simulink model "THREE_PID"  (R2019b)
settings: Solver=ode45  StartTime=0.0  StopTime=5  MaxStep=0.5  MinStep=0.00001  RelTol=0.05
model workspace: external: MAT-File workspace.mat (data not in the file)
values from neighbouring files (symbols this model uses):
  b = b+nb(i)    [genetic_pid.m]
  R = rand    [genetic_pid.m]
undefined symbols (not defined in the file or in its folder): B, F, g, GR, J1, J_rotor, k, km, kt, L, L1, L1C, M1
libraries: simulink x3, simulink_extras x3
settings Model: Creator=Kartik  LastModifiedBy=Kartik
settings SolverCC: MaxConsecutiveMinStep=20  ZeroCrossAlgorithm=Adaptive
settings DataIOCC: Refine=2
settings DebuggingCC: MaskedZcDiagnostic=none  IgnoredZcDiagnostic=none

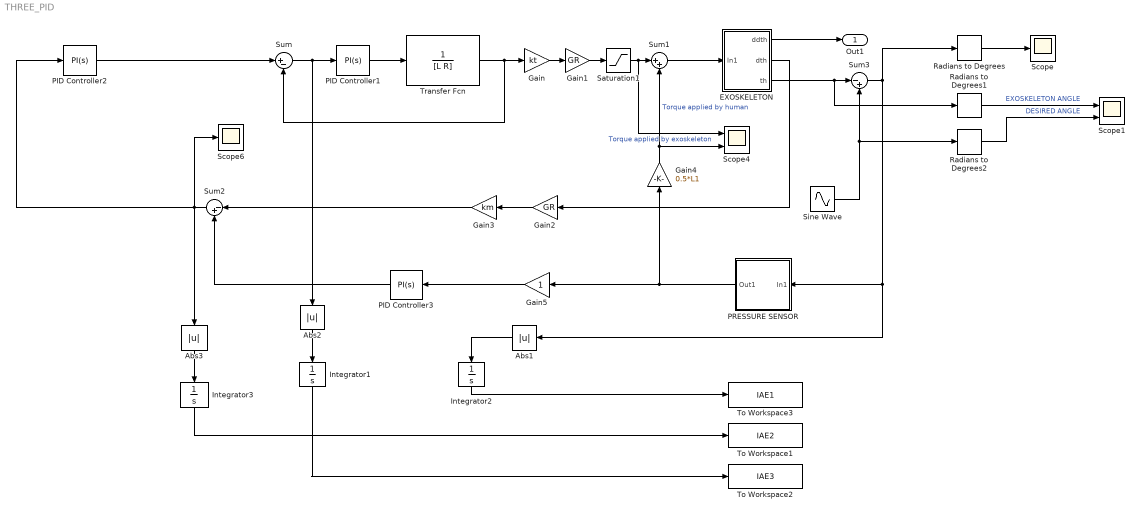
== system THREE_PID ==
  Abs1 : Abs
  Abs2 : Abs
  Abs3 : Abs
  "EXOSKELETON " : Subsystem
  Gain : Gain  Gain=kt
  Gain1 : Gain  Gain=GR
  Gain2 : Gain  Gain=GR
  Gain3 : Gain  Gain=km
  Gain4 : Gain  Gain=0.5*L1
  Gain5 : Gain
  Integrator1 : Integrator
  Integrator2 : Integrator
  Integrator3 : Integrator
  PID Controller1 : simulink/Continuous/PID Controller  Controller=PI  Form=Parallel  TimeDomain=Continuous-time  SampleTime=-1  IntegratorMethod=Forward Euler  FilterMethod=Forward Euler  ControllerParametersSource=internal  P=13.44220  I=9.960331  D=0  UseFilter=on  N=100  TunerSelectOption=Transfer Function Based (PID Tuner App)  InitialConditionSource=internal  InitialConditionForIntegrator=0  InitialConditionForFilter=0  DifferentiatorICPrevScaledInput=0  ExternalReset=none  TrackingMode=off  Kt=1  LimitOutput=off  UpperSaturationLimit=inf  LowerSaturationLimit=-inf  LinearizeAsGain=on  AntiWindupMode=none  Kb=1  POutMin=[]  POutMax=[]  IOutMin=[]  IOutMax=[]  DOutMin=[]  DOutMax=[]  NOutMin=[]  NOutMax=[]  SumOutMin=[]  SumOutMax=[]  SaturationOutMin=[]  SaturationOutMax=[]  PParamMin=[]  PParamMax=[]  IParamMin=[]  IParamMax=[]  DParamMin=[]  DParamMax=[]  NParamMin=[]  NParamMax=[]  KbParamMin=[]  KbParamMax=[]  KtParamMin=[]  KtParamMax=[]  KbOutMin=[]  KbOutMax=[]  KtOutMin=[]  KtOutMax=[]  IntegratorOutMin=[]  IntegratorOutMax=[]  FilterOutMin=[]  FilterOutMax=[]  SumI1OutMin=[]  SumI1OutMax=[]  SumI2OutMin=[]  SumI2OutMax=[]  SumI3OutMin=[]  SumI3OutMax=[]  SumI4OutMin=[]  SumI4OutMax=[]  SumDOutMin=[]  SumDOutMax=[]  DifferentiatorOutMin=[]  DifferentiatorOutMax=[]  FilterDiffOutCoefMin=[]  FilterDiffOutCoefMax=[]  ReciprocalOutMin=[]  ReciprocalOutMax=[]  SumDenOutMin=[]  SumDenOutMax=[]  SumNumOutMin=[]  SumNumOutMax=[]  DivideOutMin=[]  DivideOutMax=[]  IntegratorContinuousStateAttributes=''  IntegratorStateMustResolveToSignalObject=off  IntegratorRTWStateStorageClass=Auto  FilterContinuousStateAttributes=''  FilterStateMustResolveToSignalObject=off  FilterRTWStateStorageClass=Auto  ParallelPVariant=InternalParameters  IdealPVariant=Disabled  IVariant=InternalParameters  DVariant=Disabled  IntegratorVariant=Continuous  SatVariant=Disabled  AWVariant=Passthrough  PCopyVariant=Disabled  TRVariant=Disabled  FdbkBlocksVariant=Forward  IdealPFdbkVariant=Disabled  SatFdbkVariant=Disabled  DerivativeFilterVariant=Disabled  NVariant=Disabled  NCopyVariant=Disabled_SignalSpec  FilterICVariant=Disabled  IntegratorICVariant=InternalICs  ExternalResetVariant=Disabled  TRSumVariant=Passthrough  SumFdbkVariant=Disabled  SumVariant=Sum_PI
  PID Controller2 : simulink/Continuous/PID Controller  Controller=PI  Form=Parallel  TimeDomain=Continuous-time  SampleTime=-1  IntegratorMethod=Forward Euler  FilterMethod=Forward Euler  ControllerParametersSource=internal  P=1.611515  I=1.022319  D=0  UseFilter=on  N=100  TunerSelectOption=Transfer Function Based (PID Tuner App)  InitialConditionSource=internal  InitialConditionForIntegrator=0  InitialConditionForFilter=0  DifferentiatorICPrevScaledInput=0  ExternalReset=none  TrackingMode=off  Kt=1  LimitOutput=off  UpperSaturationLimit=inf  LowerSaturationLimit=-inf  LinearizeAsGain=on  AntiWindupMode=none  Kb=1  POutMin=[]  POutMax=[]  IOutMin=[]  IOutMax=[]  DOutMin=[]  DOutMax=[]  NOutMin=[]  NOutMax=[]  SumOutMin=[]  SumOutMax=[]  SaturationOutMin=[]  SaturationOutMax=[]  PParamMin=[]  PParamMax=[]  IParamMin=[]  IParamMax=[]  DParamMin=[]  DParamMax=[]  NParamMin=[]  NParamMax=[]  KbParamMin=[]  KbParamMax=[]  KtParamMin=[]  KtParamMax=[]  KbOutMin=[]  KbOutMax=[]  KtOutMin=[]  KtOutMax=[]  IntegratorOutMin=[]  IntegratorOutMax=[]  FilterOutMin=[]  FilterOutMax=[]  SumI1OutMin=[]  SumI1OutMax=[]  SumI2OutMin=[]  SumI2OutMax=[]  SumI3OutMin=[]  SumI3OutMax=[]  SumI4OutMin=[]  SumI4OutMax=[]  SumDOutMin=[]  SumDOutMax=[]  DifferentiatorOutMin=[]  DifferentiatorOutMax=[]  FilterDiffOutCoefMin=[]  FilterDiffOutCoefMax=[]  ReciprocalOutMin=[]  ReciprocalOutMax=[]  SumDenOutMin=[]  SumDenOutMax=[]  SumNumOutMin=[]  SumNumOutMax=[]  DivideOutMin=[]  DivideOutMax=[]  IntegratorContinuousStateAttributes=''  IntegratorStateMustResolveToSignalObject=off  IntegratorRTWStateStorageClass=Auto  FilterContinuousStateAttributes=''  FilterStateMustResolveToSignalObject=off  FilterRTWStateStorageClass=Auto  ParallelPVariant=InternalParameters  IdealPVariant=Disabled  IVariant=InternalParameters  DVariant=Disabled  IntegratorVariant=Continuous  SatVariant=Disabled  AWVariant=Passthrough  PCopyVariant=Disabled  TRVariant=Disabled  FdbkBlocksVariant=Forward  IdealPFdbkVariant=Disabled  SatFdbkVariant=Disabled  DerivativeFilterVariant=Disabled  NVariant=Disabled  NCopyVariant=Disabled_SignalSpec  FilterICVariant=Disabled  IntegratorICVariant=InternalICs  ExternalResetVariant=Disabled  TRSumVariant=Passthrough  SumFdbkVariant=Disabled  SumVariant=Sum_PI
  PID Controller3 : simulink/Continuous/PID Controller  Controller=PI  Form=Parallel  TimeDomain=Continuous-time  SampleTime=-1  IntegratorMethod=Forward Euler  FilterMethod=Forward Euler  ControllerParametersSource=internal  P=35.80372  I=4.633430  D=0  UseFilter=on  N=100  TunerSelectOption=Transfer Function Based (PID Tuner App)  InitialConditionSource=internal  InitialConditionForIntegrator=0  InitialConditionForFilter=0  DifferentiatorICPrevScaledInput=0  ExternalReset=none  TrackingMode=off  Kt=1  LimitOutput=off  UpperSaturationLimit=inf  LowerSaturationLimit=-inf  LinearizeAsGain=on  AntiWindupMode=none  Kb=1  POutMin=[]  POutMax=[]  IOutMin=[]  IOutMax=[]  DOutMin=[]  DOutMax=[]  NOutMin=[]  NOutMax=[]  SumOutMin=[]  SumOutMax=[]  SaturationOutMin=[]  SaturationOutMax=[]  PParamMin=[]  PParamMax=[]  IParamMin=[]  IParamMax=[]  DParamMin=[]  DParamMax=[]  NParamMin=[]  NParamMax=[]  KbParamMin=[]  KbParamMax=[]  KtParamMin=[]  KtParamMax=[]  KbOutMin=[]  KbOutMax=[]  KtOutMin=[]  KtOutMax=[]  IntegratorOutMin=[]  IntegratorOutMax=[]  FilterOutMin=[]  FilterOutMax=[]  SumI1OutMin=[]  SumI1OutMax=[]  SumI2OutMin=[]  SumI2OutMax=[]  SumI3OutMin=[]  SumI3OutMax=[]  SumI4OutMin=[]  SumI4OutMax=[]  SumDOutMin=[]  SumDOutMax=[]  DifferentiatorOutMin=[]  DifferentiatorOutMax=[]  FilterDiffOutCoefMin=[]  FilterDiffOutCoefMax=[]  ReciprocalOutMin=[]  ReciprocalOutMax=[]  SumDenOutMin=[]  SumDenOutMax=[]  SumNumOutMin=[]  SumNumOutMax=[]  DivideOutMin=[]  DivideOutMax=[]  IntegratorContinuousStateAttributes=''  IntegratorStateMustResolveToSignalObject=off  IntegratorRTWStateStorageClass=Auto  FilterContinuousStateAttributes=''  FilterStateMustResolveToSignalObject=off  FilterRTWStateStorageClass=Auto  ParallelPVariant=InternalParameters  IdealPVariant=Disabled  IVariant=InternalParameters  DVariant=Disabled  IntegratorVariant=Continuous  SatVariant=Disabled  AWVariant=Passthrough  PCopyVariant=Disabled  TRVariant=Disabled  FdbkBlocksVariant=Forward  IdealPFdbkVariant=Disabled  SatFdbkVariant=Disabled  DerivativeFilterVariant=Disabled  NVariant=Disabled  NCopyVariant=Disabled_SignalSpec  FilterICVariant=Disabled  IntegratorICVariant=InternalICs  ExternalResetVariant=Disabled  TRSumVariant=Passthrough  SumFdbkVariant=Disabled  SumVariant=Sum_PI
  PRESSURE SENSOR : Subsystem
  Radians to Degrees : simulink_extras/Transformations/Radians to Degrees
  Radians to Degrees1 : simulink_extras/Transformations/Radians to Degrees
  Radians to Degrees2 : simulink_extras/Transformations/Radians to Degrees
  Saturation1 : Saturate  UpperLimit=200  LowerLimit=-200
  Scope : Scope
  Scope1 : Scope  NumInputPorts=2
  Scope4 : Scope  NumInputPorts=2
  Scope6 : Scope
  Sine Wave : Sin  Amplitude=0.4  Frequency=2  SampleTime=0
  Sum : Sum  Inputs=|+-
  Sum1 : Sum  Inputs=|++
  Sum2 : Sum  Inputs=|-+
  Sum3 : Sum  Inputs=|-+
  To Workspace1 : ToWorkspace  VariableName=IAE2  SampleTime=-1
  To Workspace2 : ToWorkspace  VariableName=IAE3  SampleTime=-1
  To Workspace3 : ToWorkspace  VariableName=IAE1  SampleTime=-1
  Transfer Fcn : TransferFcn  Denominator=[L R]
  Out1 : Outport
  wires:
  PID Controller1/1 -> Transfer Fcn/1
  Sum/1 -> Abs2/1, PID Controller1/1
  PID Controller2/1 -> Sum/1
  Transfer Fcn/1 -> Gain/1, Sum/2
  Gain/1 -> Gain1/1
  "EXOSKELETON "/2(dth) -> Gain2/1
  Gain2/1 -> Gain3/1
  Gain3/1 -> Sum2/1
  "EXOSKELETON "/3(th) -> Radians to Degrees1/1, Sum3/1
  Sum3/1 -> Radians to Degrees/1, Abs1/1, PRESSURE SENSOR/1(In1)
  Gain4/1 -> Sum1/2, Scope4/2  "Torque applied by human"
  PID Controller3/1 -> Sum2/2
  "EXOSKELETON "/1(ddth) -> Out1/1
  Radians to Degrees/1 -> Scope/1
  Radians to Degrees1/1 -> Scope1/1  "EXOSKELETON ANGLE"
  Radians to Degrees2/1 -> Scope1/2  "DESIRED ANGLE"
  Abs1/1 -> Integrator2/1
  Integrator2/1 -> To Workspace3/1
  Gain5/1 -> PID Controller3/1
  PRESSURE SENSOR/1(Out1) -> Gain5/1, Gain4/1
  Gain1/1 -> Saturation1/1
  Sum1/1 -> "EXOSKELETON "/1(In1)
  Saturation1/1 -> Sum1/1, Scope4/1  "Torque applied by exoskeleton"
  Sine Wave/1 -> Sum3/2, Radians to Degrees2/1
  Sum2/1 -> Abs3/1, PID Controller2/1, Scope6/1
  Abs2/1 -> Integrator1/1
  Abs3/1 -> Integrator3/1
  Integrator1/1 -> To Workspace2/1
  Integrator3/1 -> To Workspace1/1

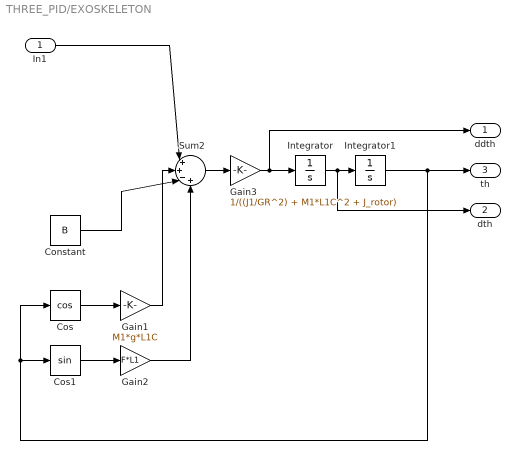
== system THREE_PID/EXOSKELETON  ==
  In1 : Inport
  Constant : Constant  Value=B
  Cos : Trigonometry  Operator=cos
  Cos1 : Trigonometry
  Gain1 : Gain  Gain=M1*g*L1C
  Gain2 : Gain  Gain=F*L1
  Gain3 : Gain  Gain=1/((J1/GR^2) + M1*L1C^2 + J_rotor)
  Integrator : Integrator
  Integrator1 : Integrator
  Sum2 : Sum  Inputs=|++-+
  ddth : Outport
  dth : Outport  Port=2
  th : Outport  Port=3
  wires:
  Integrator1/1 -> th/1, Cos1/1, Cos/1
  Cos1/1 -> Gain2/1
  Integrator/1 -> dth/1, Integrator1/1
  Gain1/1 -> Sum2/2
  Sum2/1 -> Gain3/1
  Gain3/1 -> ddth/1, Integrator/1
  Constant/1 -> Sum2/3
  Cos/1 -> Gain1/1
  In1/1 -> Sum2/1
  Gain2/1 -> Sum2/4

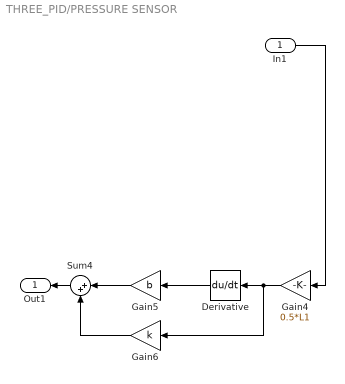
== system THREE_PID/PRESSURE SENSOR ==
  In1 : Inport
  Derivative : Derivative
  Gain4 : Gain  Gain=0.5*L1
  Gain5 : Gain  Gain=b
  Gain6 : Gain  Gain=k
  Sum4 : Sum  Inputs=|++
  Out1 : Outport
  wires:
  Gain5/1 -> Sum4/1
  Gain4/1 -> Gain6/1, Derivative/1
  Gain6/1 -> Sum4/2
  Derivative/1 -> Gain5/1
  In1/1 -> Gain4/1
  Sum4/1 -> Out1/1
